simulink model "Vehicle_Model_Controller_Aug13"  (R2021b)
settings: Solver=VariableStepAuto  StartTime=0.0  StopTime=15  FixedStep=0.015  MaxStep=0.015  RelTol=1e-3
model workspace (MAT data in the model file):
  Cx = 10000
  Dx = 2000
  Kp = 10
  understeer_gradient = 0.05
values from neighbouring files (symbols this model uses):
  a = Simulink.Parameter(1.14)    [startup.m]
  A1 = Simulink.Parameter(39.8344)    [startup.m]
  A2 = Simulink.Parameter(813.0780)    [startup.m]
  b = Simulink.Parameter(-0.03291)    [startup.m]
  B1 = Simulink.Parameter(0.000001287)    [startup.m]
  B2 = Simulink.Parameter(-0.002325)    [startup.m]
  B3 = Simulink.Parameter(3.797)    [startup.m]
  c = Simulink.Parameter(-1.14)    [startup.m]
  C1 = Simulink.Parameter(-0.000000002541)    [startup.m]
  C2 = Simulink.Parameter(0.000005279)    [startup.m]
  C3 = Simulink.Parameter(-0.003943)    [startup.m]
  C4 = Simulink.Parameter(3.634)    [startup.m]
  C_param = Simulink.Parameter([0 13757.41 21278.97 26666.02 30253.47 30313.18 30313.18])    [startup.m]
  d = Simulink.Parameter(-1.027)    [startup.m]
  driver_gain = 1    [startup.m]
  FZ_C = Simulink.Parameter([0 204.13 427.04 668.1 895.72 1124.40 1324.40])    [startup.m]
  gr = Simulink.Parameter([6.63043, 6.63043, 7.95652, 7.95652])    [startup.m]
  I = 15    [startup.m]
  inch2mm = Simulink.Parameter(25.4)    [startup.m]
  J_z = Simulink.Parameter(75)    [startup.m]
  k_limit = Simulink.Parameter(3.461)    [startup.m]
  Ku = Simulink.Parameter(0.24 / g.Value)    [startup.m]
  l = Simulink.Parameter([0.7922471, 0.7828529])    [startup.m]
  max_yaw_field = Simulink.Parameter([1.34 1.34 1.34 1.66 1.14 1.24 0.754 0.849 0.85 0.85])    [startup.m]
  min_speed_regen = Simulink.Parameter(85)    [startup.m]
  motor_efficiency = Simulink.Parameter([0.85, 0.85, 0.85, 0.85])    [startup.m]
  motor_limit_power = Simulink.Parameter([15000, 15000, 15000, 15000])    [startup.m]
  motor_limit_torque = Simulink.Parameter([-25, 25])    [startup.m]
  mu_factor = Simulink.Parameter(2/3)    [startup.m]
  P = 1    [startup.m]
  ramp_rate = 1    [startup.m]
  RE = Simulink.Parameter(0.2228169203)    [startup.m]
  s = Simulink.Parameter([0.647895, 0.62102])    [startup.m]
  S1 = Simulink.Parameter(7 * (10^(-5)))    [startup.m]
  S2 = Simulink.Parameter(-0.0038)    [startup.m]
  S3 = Simulink.Parameter(0.6535)    [startup.m]
  S4 = Simulink.Parameter(0.1061)    [startup.m]
  steer_slope = Simulink.Parameter(0.0111)    [startup.m]
  T = 0    [startup.m]
  T2F = Simulink.Parameter(single([29 29 35 35]))    [startup.m]
  tau = Simulink.Parameter(0)    [startup.m]
  time_delay = 0.022    [startup.m]
  V_target = Simulink.Parameter([0 3 6 9 12 15 18 21 25 31])    [startup.m]
undefined symbols (not defined in the file or in its folder): DiscIntNeverNeededParam
libraries: fl_lib x42, nesl_utility x37, sdl_lib x11, slpidlib x1, vehdynlibtire x1, autolibshared x1, autolibdatasheetbattery x1
(part 4 of 4)

== matlab function Vehicle_Model_Controller_Aug13/Driver Input Logic/Torque Vectoring Controller/Tire Model ==
  data: FZ input size=[1 4]; temp_vel input size=[1 6]; Fx_max output; Vg input size=[1 2]; yaw input size=1; omega input size=[1 4]; steering input size=[1 3]; FY output; s parameter; l parameter; RE parameter; A1 parameter; A2 parameter; B1 parameter; B2 parameter; B3 parameter; C1 parameter; C2 parameter; C3 parameter; C4 parameter; FZ_C parameter; C_param parameter; a parameter; b parameter; c parameter; d parameter; k_limit parameter; mu_factor parameter
function [Fx_max, FY] =  tire_model( FZ,temp_vel, Vg, yaw, omega, steering, s, l, RE, A1, A2, B1, B2, B3, C1, C2, C3, C4, FZ_C, C_param, a, b, c, d, k_limit, mu_factor)
%% Compute Steering Angles
vel = temp_vel;
acker_steer_angles = [steering(2) steering(3)];
Vx = Vg(1);
Vy = Vg(2);


%% Simulation Only
% This section is only for simulation. IGNORE THIS SECTION
% Motor Shaft Speed, m/s
%v_fl = (vel(1) * cos(acker_steer_angles(1))) + (vel(2) * sin(acker_steer_angles(1)));
%v_fr = (vel(3) * cos(acker_steer_angles(2))) + (vel(4) * sin(acker_steer_angles(2)));
%v_rl = vel(5);
%v_rr = vel(6);
%v_w = [v_fl v_fr v_rl v_rr];

% Wheel Speed, Rad/s
%omega = ((temp_SL .* abs(v_w)) + v_w) ./ RE;
%omega = v_w ./ RE;

%% Compute Tire Slip
% Velocity at each Tire
V_fl = Vg + (yaw .* [s(1) l(1)]);
V_fr = Vg + (yaw .* [-s(1) l(1)]);
V_rl = Vg + (yaw .* [s(2) -l(2)]);
V_rr = Vg + (yaw .* [-s(2) -l(2)]);

V = [V_fl V_fr V_rl V_rr];

% Individual slip angles, it blows up at low velocity
if abs(Vg(1)) > 0.1
    phi_fl = atan2(Vy + (l(1)*yaw), Vx + (s(1)*yaw));
    phi_fr = atan2(Vy + (l(1)*yaw), Vx - (s(1)*yaw));
    phi_rl = atan2(Vy - (l(2)*yaw), Vx + (s(2)*yaw));
    phi_rr = atan2(Vy - (l(2)*yaw), Vx - (s(2)*yaw));
else
    phi_fl = 0;
    phi_fr = 0;
    phi_rl = 0;
    phi_rr = 0;
end

phi = [phi_fl phi_fr phi_rl phi_rr];

% Compute Slip Angle
SA_fl = -phi_fl + acker_steer_angles(1);
SA_fr = -phi_fr + acker_steer_angles(2);
SA_rl = -phi_rl;
SA_rr = -phi_rr;

SA = [SA_fl SA_fr SA_rl SA_rr];

% Compute Slip Ratio
if abs(norm(V_fl) * cos(SA_fl)) > 0
    SL_fl = ((RE * omega(1))/(norm(V_fl) * cos(SA_fl))) - 1;
else
    SL_fl = 0;
end

if abs(norm(V_fl) * cos(SA_fl)) > 0
    SL_fr = ((RE * omega(2))/(norm(V_fr) * cos(SA_fr))) - 1;
else
    SL_fr = 0;
end

if abs(norm(V_fl) * cos(SA_fl)) > 0
    SL_rl = ((RE * omega(3))/(norm(V_rl) * cos(SA_rl))) - 1;
else
    SL_rl = 0;
end

if abs(norm(V_fl) * cos(SA_fl)) > 0
    SL_rr = ((RE * omega(4))/(norm(V_rr) * cos(SA_rr))) - 1;
else
    SL_rr = 0;
end


% This line is commented out only for simulation. On the vehicle, this
% line is to be included.
SL = [SL_fl SL_fr SL_rl SL_rr];

%% Non Dimensional Tire Model
% Basic Coefficients
kx = (A1 .* (FZ)) + A2;
C = pchip(FZ_C, C_param, abs(FZ));
mu_x = ((B1 .* (FZ.^2)) + (B2 .* (FZ)) + B3);
mu_y = ((C1 .* (FZ.^3)) + (C2 .* (FZ.^2)) + (C3 .* (FZ)) + C4);

% Normalized Slip Ratio, Slip Angle
s_bar = (kx .* SL) ./ (mu_x .* FZ);

% C is a function of FZ, but it is not an analytical expression
a_bar = (C .* tan(SA)) ./ (mu_y .* FZ);

% Combined Slip Model Parameters
n0 = (C .* mu_x) ./ (kx .* mu_y);
k = sqrt(s_bar.^2 + a_bar.^2);
n = [1 1 1 1];

for i = 1:4
    if abs(k(i)) <= (2*pi)
       n = (0.5 .* (1 + n0)) - (0.5 .* cos(k/2) .* (1 - n0));
    end
end

% Compute R, the bridge between tire slip and tire forces
R = (a .* exp(b .* k)) + (c .* exp(d .* k));

% Find FX & FY, denominator blows up at no slip
FY = [0 0 0 0];
FX = [0 0 0 0];

for i = 1:4
   if ~((abs(sqrt(SL(i).^2 + ((n(i).^2) .* (tan(SA(i))).^2))) < 0.001 && norm([Vx Vy]) < 3))
       FX(i) = (mu_x(i) .* FZ(i) .* R(i) .* SL(i)) ./ (sqrt(SL(i).^2 + ((n(i).^2) .* (tan(SA(i))).^2)));
       FY(i) = (n(i) .* R(i) .* tan(SA(i)) .* mu_y(i) .* FZ(i)) ./ (sqrt(SL(i).^2 + ((n(i).^2) .* (tan(SA(i))).^2)));
   end
end


%% Max Longitudinal Force
% Constant during runtime
R_max = [1 1 1 1] .* (a .* exp(b .* k_limit)) + (c .* exp(d .* k_limit));
n_max = [1 1 1 1];
if abs(k(i)) <= (2*pi)
   n_max = [1 1 1 1] .* (0.5 .* (1 + n0)) - (0.5 .* cos(k_limit/2) .* (1 - n0));
end

s_bar_max = [0 0 0 0];

for i = 1:4
    if k_limit > abs(a_bar(i))
        s_bar_max(i) = sqrt(k_limit^2 - a_bar(i)^2);
    end
end

SL_max = (s_bar_max .* mu_x .* FZ) ./ (kx);

Fx_max = (mu_x .* FZ .* R_max .* SL_max) ./ (sqrt(SL_max.^2 + ((n_max.^2) .* (tan(SA)).^2)));

%% Compare FY Calculations
% Incomplete, or will not be implemented
FY = FY .* mu_factor;
end

== matlab function Vehicle_Model_Controller_Aug13/Driver Input Logic/Torque Vectoring Controller/Brake Model ==
  data: brake_pressure input size=[1 4]; T_brake output size=[1 4]; Vx input size=1; brakecoeff parameter size=[1 4]
function T_brake = brake_model(brake_pressure, Vx, brakecoeff)
%% Inputs
% brake_pressure_front     [MPa]
% brake_pressure_rear      [MPa]
% omega_wheel_RL           [rad/s]

%% Outputs
% T_Brake                  [Nm][1x4]
%    T_Brake_FL
%    T_Brake_FR
%    T_Brake_RL
%    T_Brake_RR


%% Compute
T_brake = zeros(1, 4);

if abs(Vx) > 5
   T_brake = -brakecoeff .* sign(Vx) .* brake_pressure;
end

end
